simulink model "ECE3331LAB2SLX1"  (R2018a)
settings: Solver=FixedStepDiscrete  StartTime=0.0  StopTime=10.0  FixedStep=0.01  RelTol=1e-3
settings Model: Creator=zshang3  LastModifiedBy=zshang3

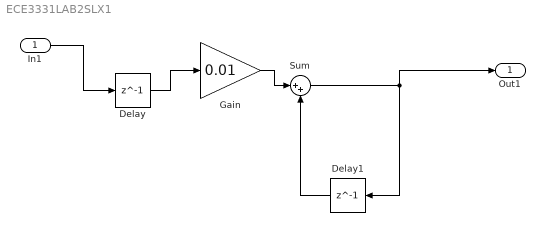
== system ECE3331LAB2SLX1 ==
  In1 : Inport
  Delay : Delay  DelayLength=1  InitialCondition=0
  Delay1 : Delay  DelayLength=1  InitialCondition=0
  Gain : Gain  Gain=0.01
  Sum : Sum  Inputs=|++
  Out1 : Outport  SignalName=Y(z)
  wires:
  In1/1 -> Delay/1
  Delay/1 -> Gain/1
  Gain/1 -> Sum/1
  Sum/1 -> Out1/1, Delay1/1
  Delay1/1 -> Sum/2
